simulink model "nuri3s_feedforward"  (R2024b)
settings: Solver=VariableStepAuto  StartTime=0.0  StopTime=5  RelTol=1e-3
undefined symbols (not defined in the file): q0, qe, qn, robot
libraries: robotmaniplib x2, robotcorelib x1
settings Model: Creator=user  LastModifiedBy=변재형

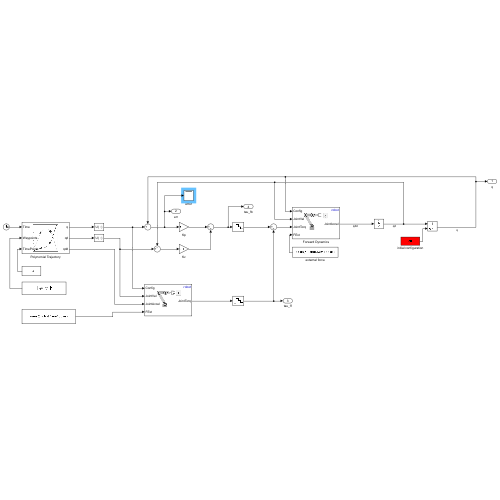
[thumbnail: Simulink's stored preview of the top-level diagram]
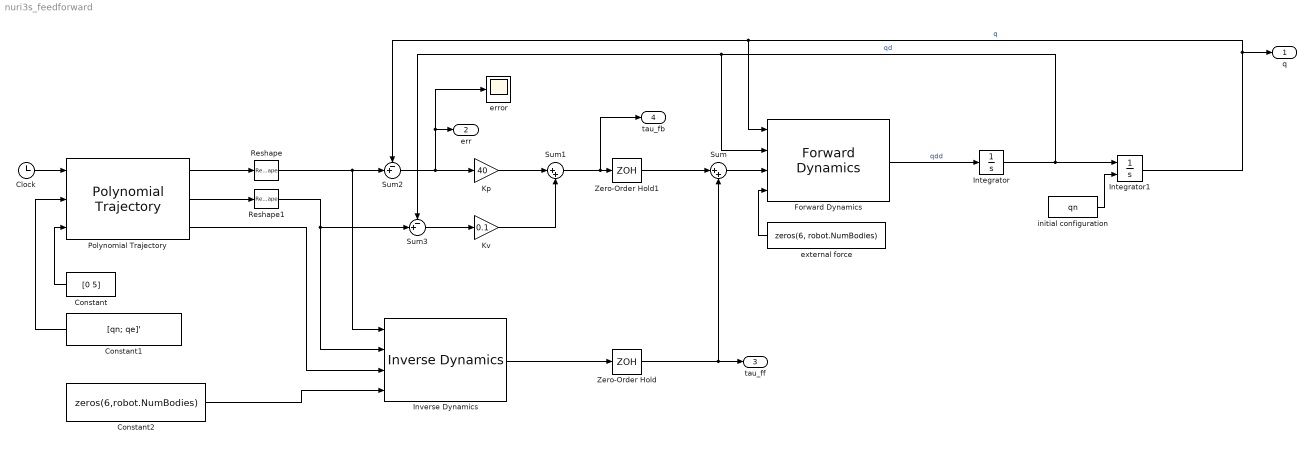
== system nuri3s_feedforward ==
  Clock : Clock
  Constant : Constant  Value=[0 5]
  Constant1 : Constant  Value=[qn; qe]'
  Constant2 : Constant  Value=zeros(6,robot.NumBodies)
  Forward Dynamics : robotmaniplib/Forward Dynamics  RigidBodyTree=robot  SimulateUsing=Interpreted execution
  Integrator : Integrator
  Integrator1 : Integrator  InitialConditionSource=external  InitialCondition=q0
  Inverse Dynamics : robotmaniplib/Inverse Dynamics  RigidBodyTree=robot  SimulateUsing=Interpreted execution
  Kp : Gain  Gain=40
  Kv : Gain  Gain=0.1
  Polynomial Trajectory : robotcorelib/Polynomial Trajectory  WaypointSource=External  Waypoints=[ 0, 2, 1, 5, 0; -1, 3, 1, 4, 4 ]  TimePoints=[ 0, 1, 2, 3, 4 ]  TimeInterval=[ 1, 4 ]  Method=Quintic Polynomial  ParameterSource=Internal  VelocityBoundaryCondition=zeros( 6, 2 )  AccelerationBoundaryCondition=zeros( 6, 2 )  SimulateUsing=Interpreted execution
  Reshape : Reshape
  Reshape1 : Reshape
  Sum : Sum  Inputs=|++
  Sum1 : Sum  Inputs=|++
  Sum2 : Sum  Inputs=-+|
  Sum3 : Sum  Inputs=-+|
  Zero-Order Hold : ZeroOrderHold  SampleTime=0.01
  Zero-Order Hold1 : ZeroOrderHold  SampleTime=0.002
  error : Scope
  external force : Constant  Value=zeros(6, robot.NumBodies)
  initial configuration : Constant  Value=qn
  q : Outport
  err : Outport  Port=2
  tau_ff : Outport  Port=3
  tau_fb : Outport  Port=4
  wires:
  Forward Dynamics/1 -> Integrator/1  "qdd"
  Integrator/1 -> Forward Dynamics/2, Sum3/1, Integrator1/1  "qd"
  Integrator1/1 -> Forward Dynamics/1, Sum2/1, q/1  "q"
  external force/1 -> Forward Dynamics/4
  Clock/1 -> Polynomial Trajectory/1
  Polynomial Trajectory/1 -> Reshape/1
  Polynomial Trajectory/2 -> Reshape1/1
  Constant/1 -> Polynomial Trajectory/3
  Constant1/1 -> Polynomial Trajectory/2
  Constant2/1 -> Inverse Dynamics/4
  Polynomial Trajectory/3 -> Inverse Dynamics/3
  Reshape1/1 -> Sum3/2, Inverse Dynamics/2
  Reshape/1 -> Sum2/2, Inverse Dynamics/1
  Inverse Dynamics/1 -> Zero-Order Hold/1
  Zero-Order Hold/1 -> Sum/2, tau_ff/1
  Sum/1 -> Forward Dynamics/3
  Sum1/1 -> tau_fb/1, Zero-Order Hold1/1
  Kp/1 -> Sum1/1
  Kv/1 -> Sum1/2
  Sum3/1 -> Kv/1
  Sum2/1 -> Kp/1, error/1, err/1
  Zero-Order Hold1/1 -> Sum/1
  initial configuration/1 -> Integrator1/2
